simulink model "Model"  (R2021a)
settings: Solver=ode4  StartTime=0.0  StopTime=inf  FixedStep=Ts  RelTol=1e-3
PreLoadFcn:
  | filepath  = fileparts(get_param(bdroot, 'FileName'))
  | cd(filepath);
values from neighbouring files (symbols this model uses):
  A_GRotation = [0 0 0]    [Parameter_PX4.m]
  ACC_UserFault = 0    [Parameter_PX4.m]
  ACCDrift = 0.0    (= 0)    [Parameter_PX4.m]
  ACCNoise = 1.0    (= 1)    [Parameter_PX4.m]
  accnoisegain = 0    [Parameter_PX4.m]
  ACCScale = 1.0    (= 1)    [Parameter_PX4.m]
  BaroNoise = 1.0    (= 1)    [Parameter_PX4.m]
  GyroDrift = 0.0    (= 0)    [Parameter_PX4.m]
  GyroNoise = 1.0    (= 1)    [Parameter_PX4.m]
  GyroScale = 1.0    (= 1)    [Parameter_PX4.m]
  MagDrift = 0.0    (= 0)    [Parameter_PX4.m]
  MagNoise = 1.0    (= 1)    [Parameter_PX4.m]
  MagRotation = [0 0 0]    [Parameter_PX4.m]
  MagScale = 1.0    (= 1)    [Parameter_PX4.m]
  ModelInit_GroundSlope = [0,0]    [Parameter_PX4.m]
  ModelInit_RPM = 0    [Parameter_PX4.m]
  ModelParam_envAltitude = -100    [Parameter_PX4.m]
  ModelParam_GlobalNoiseGainSwitch = 0.4    [Parameter_PX4.m]
  ModelParam_GPSEphFinal = 0.3    [Parameter_PX4.m]
  ModelParam_GPSEpvFinal = 0.4    [Parameter_PX4.m]
  ModelParam_GPSFix3DFix = 3    [Parameter_PX4.m]
  ModelParam_GPSSatsVisible = 10    [Parameter_PX4.m]
  ModelParam_motorCr = 842.1    [Parameter_PX4.m]
  ModelParam_motorJm = 0.0001287    [Parameter_PX4.m]
  ModelParam_motorMinThr = 0.05    [Parameter_PX4.m]
  ModelParam_motorT = 0.0214    [Parameter_PX4.m]
  ModelParam_motorWb = 22.83    [Parameter_PX4.m]
  ModelParam_noiseBaroCoupleWithSpeed = 0    [Parameter_PX4.m]
  ModelParam_noiseUpperWindBodyRatio = 0    [Parameter_PX4.m]
  ModelParam_rotorCm = 2.783e-07    [Parameter_PX4.m]
  ModelParam_rotorCt = 1.681e-05    [Parameter_PX4.m]
  ModelParam_uavCCm = [0.0035 0.0039 0.0034]    [Parameter_PX4.m]
  ModelParam_uavCd = 0.055    [Parameter_PX4.m]
  ModelParam_uavDearo = 0.12    [Parameter_PX4.m]
  ModelParam_uavMass = 1.515    [Parameter_PX4.m]
  ModelParam_uavR = 0.225    [Parameter_PX4.m]
  ModelParam_uavType = int8(3)    [Parameter_PX4.m]
  MyNoiseGain = [2.5;3;4].*3    [Parameter_PX4.m]
  PWMNoiseGain = [10;15;3]    [Parameter_PX4.m]
  TemperatureConstant = 25.0    (= 25)    [Parameter_PX4.m]
  Ts = 1/2000    (= 0.0005)    [Parameter_PX4.m]
  TypeMotorAngMatrix = [     [pi/3 pi -pi/3 0 0 0 0 0];     [pi/3 pi -pi/3 0 0 0 0 0];     [pi/4 pi/4+pi pi/4+3*pi/2 pi/4+pi/2 0 0 0 0];     [pi/2 3*pi/2 0 pi 0 0 0 0];     [pi/2 3/2*pi 3/2*pi+pi/3 pi/2+pi/3 pi/2-pi/3 3/2*pi-pi/3 0 0];     [0 pi pi+pi/3 pi/3 -pi/3 pi-pi/3 0 0];     [pi/3 pi/3 pi pi -pi/3 -pi/3 0 0];     [pi/8 pi+pi/8 pi/8+pi/4 pi-pi/8 -pi/8 3/2*pi-pi/8 3/2*pi+pi/8 pi/2+pi/8];     [0 pi pi/4 3/4*pi -pi/4 ...(+86 chars)    [Parameter_PX4.m]
  TypeMotorDirMatrix = [     [-1 -1 -1 0 0 0 0 0];     [1 1 1 0 0 0 0 0];     [-1 -1 1 1 0 0 0 0];     [-1 -1 1 1 0 0 0 0];     [1 -1 1 -1 -1 1 0 0];     [1 -1 1 -1 -1 1 0 0];     [1 -1 1 -1 1 -1 0 0];     [1 1 -1 -1 -1 -1 1 1];     [1 1 -1 -1 -1 -1 1 1];     [-1 1 -1 1 -1 1 -1 1]; ]'    [Parameter_PX4.m]
  TypeMotorNonVector = int8([3;3;4;4;6;6;6;8;8;8])    [Parameter_PX4.m]
undefined symbols (not defined in the file or in its folder): Earth, ModelParam_GPSEpvInitial, ModelParam_GPSEpvTimeConstant, ModelParam_noiseGPSSampTime, ModelParam_noisePowerIMU, ModelParam_noisePowerOffGainAccel, ModelParam_noisePowerOffGainAccelZ, ModelParam_noisePowerOffGainGyro, ModelParam_noisePowerOffGainGyroZ, ModelParam_noisePowerOffGainMag, ModelParam_noisePowerOffGainMagZ, ModelParam_noisePowerOnGainAccel, ModelParam_noisePowerOnGainAccelZ, ModelParam_noisePowerOnGainGyro, ModelParam_noisePowerOnGainGyroZ, ModelParam_noisePowerOnGainMag, ModelParam_noisePowerOnGainMagZ, ModelParam_noiseUpperGPS, ModelParam_timeSamp, Newton, Raphson, WGS84
libraries: simulink x11, sharedtransform x7, aerolibutil x4, aerolibtransform2 x4, aerolibasang x3, simulink_extras x2, etargetslib x2, aerolibatmos2 x2, shared6dof x1, aerolibconvert2 x1, aerolibobsolete x1, aerolibnav x1
(part 2 of 3)

== system Model/Motor Model/MotorNonlinearDynamic2 ==
  Wb : Inport
  Cr : Inport  Port=2
  motorT : Inport  Port=3
  ModelInit_RPM : Inport  Port=4
  PWM : Inport  Port=5
  Minimum Throttle Cutoff : simulink/Logic and Bit Operations/Compare To Constant  relop=>=  const=ModelParam_motorMinThr  OutDataTypeStr=uint8
  Motor_Dynamics : Subsystem  TreatAsAtomicUnit=on
  Motor_Dynamics_backup : StateSpace  Commented=on  A=-1/ModelParam_motorT  C=1/ModelParam_motorT  D=0  InitialCondition=ModelInit_RPM*ModelParam_motorT
  Product : Product
  Product1 : Product
  Signal_Saturation : Saturate  UpperLimit=0.95  LowerLimit=0
  Sum1 : Sum  Inputs=++|
  radW : Outport  VectorParamsAs1DForOutWhenUnconnected=off
  wires:
  ModelInit_RPM/1 -> Motor_Dynamics/2(ModelInit_RPM)
  motorT/1 -> Motor_Dynamics/3(motorT)
  Cr/1 -> Product1/1
  Minimum Throttle Cutoff/1 -> Product/2
  Wb/1 -> Sum1/1
  Sum1/1 -> Product/1
  Product1/1 -> Sum1/2
  Signal_Saturation/1 -> Minimum Throttle Cutoff/1, Product1/2
  Product/1 -> Motor_Dynamics/1(motor_rate_d)
  Motor_Dynamics/1(motor_rate_act) -> radW/1
  PWM/1 -> Signal_Saturation/1

== system Model/Motor Model/MotorNonlinearDynamic3 ==
  Wb : Inport
  Cr : Inport  Port=2
  motorT : Inport  Port=3
  ModelInit_RPM : Inport  Port=4
  PWM : Inport  Port=5
  Minimum Throttle Cutoff : simulink/Logic and Bit Operations/Compare To Constant  relop=>=  const=ModelParam_motorMinThr  OutDataTypeStr=uint8
  Motor_Dynamics : Subsystem  TreatAsAtomicUnit=on
  Motor_Dynamics_backup : StateSpace  Commented=on  A=-1/ModelParam_motorT  C=1/ModelParam_motorT  D=0  InitialCondition=ModelInit_RPM*ModelParam_motorT
  Product : Product
  Product1 : Product
  Signal_Saturation : Saturate  UpperLimit=0.95  LowerLimit=0
  Sum1 : Sum  Inputs=++|
  radW : Outport  VectorParamsAs1DForOutWhenUnconnected=off
  wires:
  PWM/1 -> Signal_Saturation/1
  Motor_Dynamics/1(motor_rate_act) -> radW/1
  Product/1 -> Motor_Dynamics/1(motor_rate_d)
  Signal_Saturation/1 -> Product1/2, Minimum Throttle Cutoff/1
  Product1/1 -> Sum1/2
  Sum1/1 -> Product/1
  Wb/1 -> Sum1/1
  Minimum Throttle Cutoff/1 -> Product/2
  Cr/1 -> Product1/1
  motorT/1 -> Motor_Dynamics/3(motorT)
  ModelInit_RPM/1 -> Motor_Dynamics/2(ModelInit_RPM)

== system Model/Motor Model/MotorNonlinearDynamic4 ==
  Wb : Inport
  Cr : Inport  Port=2
  motorT : Inport  Port=3
  ModelInit_RPM : Inport  Port=4
  PWM : Inport  Port=5
  Minimum Throttle Cutoff : simulink/Logic and Bit Operations/Compare To Constant  relop=>=  const=ModelParam_motorMinThr  OutDataTypeStr=uint8
  Motor_Dynamics : Subsystem  TreatAsAtomicUnit=on
  Motor_Dynamics_backup : StateSpace  Commented=on  A=-1/ModelParam_motorT  C=1/ModelParam_motorT  D=0  InitialCondition=ModelInit_RPM*ModelParam_motorT
  Product : Product
  Product1 : Product
  Signal_Saturation : Saturate  UpperLimit=0.95  LowerLimit=0
  Sum1 : Sum  Inputs=++|
  radW : Outport  VectorParamsAs1DForOutWhenUnconnected=off
  wires:
  ModelInit_RPM/1 -> Motor_Dynamics/2(ModelInit_RPM)
  motorT/1 -> Motor_Dynamics/3(motorT)
  Cr/1 -> Product1/1
  Minimum Throttle Cutoff/1 -> Product/2
  Wb/1 -> Sum1/1
  Sum1/1 -> Product/1
  Product1/1 -> Sum1/2
  Signal_Saturation/1 -> Minimum Throttle Cutoff/1, Product1/2
  Product/1 -> Motor_Dynamics/1(motor_rate_d)
  Motor_Dynamics/1(motor_rate_act) -> radW/1
  PWM/1 -> Signal_Saturation/1

== system Model/Motor Model/MotorNonlinearDynamic5 ==
  Wb : Inport
  Cr : Inport  Port=2
  motorT : Inport  Port=3
  ModelInit_RPM : Inport  Port=4
  PWM : Inport  Port=5
  Minimum Throttle Cutoff : simulink/Logic and Bit Operations/Compare To Constant  relop=>=  const=ModelParam_motorMinThr  OutDataTypeStr=uint8
  Motor_Dynamics : Subsystem  TreatAsAtomicUnit=on
  Motor_Dynamics_backup : StateSpace  Commented=on  A=-1/ModelParam_motorT  C=1/ModelParam_motorT  D=0  InitialCondition=ModelInit_RPM*ModelParam_motorT
  Product : Product
  Product1 : Product
  Signal_Saturation : Saturate  UpperLimit=0.95  LowerLimit=0
  Sum1 : Sum  Inputs=++|
  radW : Outport  VectorParamsAs1DForOutWhenUnconnected=off
  wires:
  PWM/1 -> Signal_Saturation/1
  Motor_Dynamics/1(motor_rate_act) -> radW/1
  Product/1 -> Motor_Dynamics/1(motor_rate_d)
  Signal_Saturation/1 -> Product1/2, Minimum Throttle Cutoff/1
  Product1/1 -> Sum1/2
  Sum1/1 -> Product/1
  Wb/1 -> Sum1/1
  Minimum Throttle Cutoff/1 -> Product/2
  Cr/1 -> Product1/1
  motorT/1 -> Motor_Dynamics/3(motorT)
  ModelInit_RPM/1 -> Motor_Dynamics/2(ModelInit_RPM)

== system Model/Motor Model/MotorNonlinearDynamic6 ==
  Wb : Inport
  Cr : Inport  Port=2
  motorT : Inport  Port=3
  ModelInit_RPM : Inport  Port=4
  PWM : Inport  Port=5
  Minimum Throttle Cutoff : simulink/Logic and Bit Operations/Compare To Constant  relop=>=  const=ModelParam_motorMinThr  OutDataTypeStr=uint8
  Motor_Dynamics : Subsystem  TreatAsAtomicUnit=on
  Motor_Dynamics_backup : StateSpace  Commented=on  A=-1/ModelParam_motorT  C=1/ModelParam_motorT  D=0  InitialCondition=ModelInit_RPM*ModelParam_motorT
  Product : Product
  Product1 : Product
  Signal_Saturation : Saturate  UpperLimit=0.95  LowerLimit=0
  Sum1 : Sum  Inputs=++|
  radW : Outport  VectorParamsAs1DForOutWhenUnconnected=off
  wires:
  ModelInit_RPM/1 -> Motor_Dynamics/2(ModelInit_RPM)
  motorT/1 -> Motor_Dynamics/3(motorT)
  Cr/1 -> Product1/1
  Minimum Throttle Cutoff/1 -> Product/2
  Wb/1 -> Sum1/1
  Sum1/1 -> Product/1
  Product1/1 -> Sum1/2
  Signal_Saturation/1 -> Minimum Throttle Cutoff/1, Product1/2
  Product/1 -> Motor_Dynamics/1(motor_rate_d)
  Motor_Dynamics/1(motor_rate_act) -> radW/1
  PWM/1 -> Signal_Saturation/1

== system Model/Motor Model/MotorNonlinearDynamic7 ==
  Wb : Inport
  Cr : Inport  Port=2
  motorT : Inport  Port=3
  ModelInit_RPM : Inport  Port=4
  PWM : Inport  Port=5
  Minimum Throttle Cutoff : simulink/Logic and Bit Operations/Compare To Constant  relop=>=  const=ModelParam_motorMinThr  OutDataTypeStr=uint8
  Motor_Dynamics : Subsystem  TreatAsAtomicUnit=on
  Motor_Dynamics_backup : StateSpace  Commented=on  A=-1/ModelParam_motorT  C=1/ModelParam_motorT  D=0  InitialCondition=ModelInit_RPM*ModelParam_motorT
  Product : Product
  Product1 : Product
  Signal_Saturation : Saturate  UpperLimit=0.95  LowerLimit=0
  Sum1 : Sum  Inputs=++|
  radW : Outport  VectorParamsAs1DForOutWhenUnconnected=off
  wires:
  PWM/1 -> Signal_Saturation/1
  Motor_Dynamics/1(motor_rate_act) -> radW/1
  Product/1 -> Motor_Dynamics/1(motor_rate_d)
  Signal_Saturation/1 -> Product1/2, Minimum Throttle Cutoff/1
  Product1/1 -> Sum1/2
  Sum1/1 -> Product/1
  Wb/1 -> Sum1/1
  Minimum Throttle Cutoff/1 -> Product/2
  Cr/1 -> Product1/1
  motorT/1 -> Motor_Dynamics/3(motorT)
  ModelInit_RPM/1 -> Motor_Dynamics/2(ModelInit_RPM)

== system Model/Motor Model/MotorNonlinearDynamic8 ==
  Wb : Inport
  Cr : Inport  Port=2
  motorT : Inport  Port=3
  ModelInit_RPM : Inport  Port=4
  PWM : Inport  Port=5
  Minimum Throttle Cutoff : simulink/Logic and Bit Operations/Compare To Constant  relop=>=  const=ModelParam_motorMinThr  OutDataTypeStr=uint8
  Motor_Dynamics : Subsystem  TreatAsAtomicUnit=on
  Motor_Dynamics_backup : StateSpace  Commented=on  A=-1/ModelParam_motorT  C=1/ModelParam_motorT  D=0  InitialCondition=ModelInit_RPM*ModelParam_motorT
  Product : Product
  Product1 : Product
  Signal_Saturation : Saturate  UpperLimit=0.95  LowerLimit=0
  Sum1 : Sum  Inputs=++|
  radW : Outport  VectorParamsAs1DForOutWhenUnconnected=off
  wires:
  ModelInit_RPM/1 -> Motor_Dynamics/2(ModelInit_RPM)
  motorT/1 -> Motor_Dynamics/3(motorT)
  Cr/1 -> Product1/1
  Minimum Throttle Cutoff/1 -> Product/2
  Wb/1 -> Sum1/1
  Sum1/1 -> Product/1
  Product1/1 -> Sum1/2
  Signal_Saturation/1 -> Minimum Throttle Cutoff/1, Product1/2
  Product/1 -> Motor_Dynamics/1(motor_rate_d)
  Motor_Dynamics/1(motor_rate_act) -> radW/1
  PWM/1 -> Signal_Saturation/1

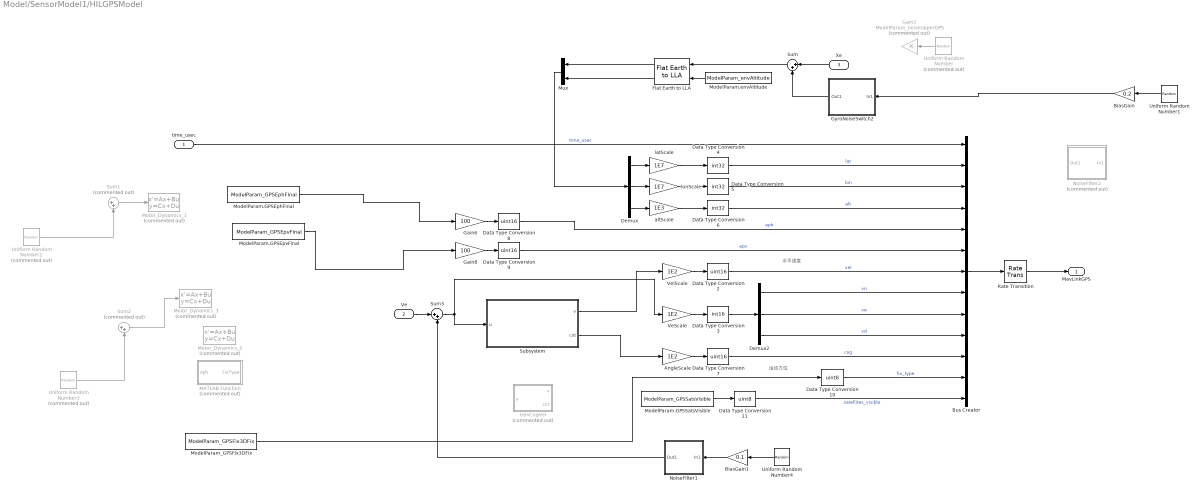
== system Model/SensorModel1/HILGPSModel ==
  note: 水平速度
  note: 运动方位
  time_usec : Inport
  Ve : Inport  Port=2
  Xe : Inport  Port=3
  AngleScale : Gain  Gain=1E2
  BiasGain : Gain  Gain=0.2
  BiasGain1 : Gain  Gain=0.1
  Bus Creator : BusCreator  Inputs=13  OutDataTypeStr=Bus: MavLinkGPS  NonVirtualBus=on
  Data Type Conversion10 : DataTypeConversion  OutDataTypeStr=uint8  RndMeth=Round
  Data Type Conversion11 : DataTypeConversion  OutDataTypeStr=uint8  RndMeth=Round
  Data Type Conversion{2,7..9} (4 alike) : DataTypeConversion  OutDataTypeStr=uint16  RndMeth=Round
  Data Type Conversion3 : DataTypeConversion  OutDataTypeStr=int16  RndMeth=Round
  Data Type Conversion4 : DataTypeConversion  OutDataTypeStr=int32  RndMeth=Round
  Data Type Conversion5 : DataTypeConversion  OutDataTypeStr=int32  RndMeth=Round
  Data Type Conversion6 : DataTypeConversion  OutDataTypeStr=int32  RndMeth=Round
  Demux : Demux  Outputs=3
  Demux2 : Demux  Outputs=3
  Flat Earth to LLA : aerolibtransform2/Flat Earth to LLA  units=Metric (MKS)  ptype=Earth (WGS84)  F=1/298.257223563  R=6378137  refPosPort=off  LL0=ModelParam_GPSLatLong  psi=0
  Gain2 : Gain  Commented=on  Gain=ModelParam_noiseUpperGPS
  Gain6 : Gain  Gain=100
  Gain8 : Gain  Gain=100
  GenCogVel : MATLAB Function  Commented=on  TreatAsAtomicUnit=on
  GyroNoiseSwitch2 : Subsystem
  MATLAB Function : MATLAB Function  Commented=on  TreatAsAtomicUnit=on
  ModelParam.GPSEphFinal : Constant  Value=ModelParam_GPSEphFinal
  ModelParam.GPSEpvFinal : Constant  Value=ModelParam_GPSEpvFinal
  ModelParam.GPSSatsVisible : Constant  Value=ModelParam_GPSSatsVisible
  ModelParam.envAltitude : Constant  Value=ModelParam_envAltitude
  ModelParam_GPSFix3DFix : Constant  Value=ModelParam_GPSFix3DFix
  Motor_Dynamics_1 : StateSpace  Commented=on  A=-1/0.2  C=1/0.2  D=0  InitialCondition=20*0.2
  Motor_Dynamics_2 : StateSpace  Commented=on  A=-1/ModelParam_GPSEpvTimeConstant  C=1/ModelParam_GPSEpvTimeConstant  D=0  InitialCondition=ModelParam_GPSEpvInitial*ModelParam_GPSEpvTimeConstant
  Motor_Dynamics_3 : StateSpace  Commented=on  A=-1/0.2  C=1/0.2  D=0  InitialCondition=20*0.2
  Mux : Mux  Inputs=2
  NoiseFilter1 : Subsystem
  NoiseFilter2 : Subsystem  Commented=on
  Rate Transition : RateTransition  OutPortSampleTime=0.05
  Subsystem : Subsystem
  Sum : Sum  Inputs=|++
  Sum1 : Sum  Commented=on  Inputs=|++
  Sum2 : Sum  Commented=on  Inputs=|++
  Sum3 : Sum  Inputs=|++
  Uniform Random Number : UniformRandomNumber  Commented=on  Minimum=[-1,-1,-3]  Maximum=[1,1,3]  Seed=[14524,7875,698]  SampleTime=ModelParam_timeSamp
  Uniform Random Number1 : UniformRandomNumber  Maximum=[1,1,2]  Seed=[1452,787,69]  SampleTime=0.05
  Uniform Random Number2 : UniformRandomNumber  Commented=on  Minimum=-0.01  Maximum=0.01  Seed=4345454  SampleTime=ModelParam_noiseGPSSampTime
  Uniform Random Number3 : UniformRandomNumber  Commented=on  Seed=3244333  SampleTime=ModelParam_noiseGPSSampTime
  Uniform Random Number4 : UniformRandomNumber  Minimum=[-1,-1,-2]  Maximum=[1,1,2]  Seed=[5445,45433,33433]  SampleTime=0.05
  VeScale : Gain  Gain=1E2
  VelScale : Gain  Gain=1E2
  altScale : Gain  Gain=1E3
  latScale : Gain  Gain=1E7
  lonScale : Gain  Gain=1E7
  MavLinkGPS : Outport  VectorParamsAs1DForOutWhenUnconnected=off
  wires:
  Data Type Conversion8/1 -> Bus Creator/5  "eph"
  Gain8/1 -> Data Type Conversion9/1
  Gain6/1 -> Data Type Conversion8/1
  Data Type Conversion9/1 -> Bus Creator/6  "epv"
  time_usec/1 -> Bus Creator/1  "time_usec"
  latScale/1 -> Data Type Conversion4/1
  lonScale/1 -> Data Type Conversion5/1
  altScale/1 -> Data Type Conversion6/1
  Data Type Conversion4/1 -> Bus Creator/2  "lat"
  Data Type Conversion5/1 -> Bus Creator/3  "lon"
  Data Type Conversion6/1 -> Bus Creator/4  "alt"
  Demux2/1 -> Bus Creator/8  "vn"
  Demux2/2 -> Bus Creator/9  "ve"
  Demux2/3 -> Bus Creator/10  "vd"
  VeScale/1 -> Data Type Conversion3/1
  Data Type Conversion3/1 -> Demux2/1
  VelScale/1 -> Data Type Conversion2/1
  Data Type Conversion2/1 -> Bus Creator/7  "vel"
  AngleScale/1 -> Data Type Conversion7/1
  Data Type Conversion7/1 -> Bus Creator/11  "cog"
  Data Type Conversion11/1 -> Bus Creator/13  "satellites_visible"
  Data Type Conversion10/1 -> Bus Creator/12  "fix_type"
  ModelParam.GPSSatsVisible/1 -> Data Type Conversion11/1
  Flat Earth to LLA/2 -> Mux/2
  ModelParam.envAltitude/1 -> Flat Earth to LLA/2
  Xe/1 -> Sum/1
  Flat Earth to LLA/1 -> Mux/1
  Demux/1 -> latScale/1
  Demux/2 -> lonScale/1
  Demux/3 -> altScale/1
  Uniform Random Number/1 -> Gain2/1
  Sum/1 -> Flat Earth to LLA/1
  Uniform Random Number1/1 -> BiasGain/1
  BiasGain/1 -> GyroNoiseSwitch2/1(In1)
  Mux/1 -> Demux/1
  ModelParam.GPSEphFinal/1 -> Gain6/1
  Sum2/1 -> Motor_Dynamics_3/1
  ModelParam_GPSFix3DFix/1 -> Data Type Conversion10/1
  Ve/1 -> Sum3/1
  GyroNoiseSwitch2/1(Out1) -> Sum/2
  BiasGain1/1 -> NoiseFilter1/1(In1)
  Uniform Random Number4/1 -> BiasGain1/1
  Sum1/1 -> Motor_Dynamics_1/1
  Uniform Random Number2/1 -> Sum1/2
  Uniform Random Number3/1 -> Sum2/2
  ModelParam.GPSEpvFinal/1 -> Gain8/1
  Sum3/1 -> Subsystem/1(u), VeScale/1
  NoiseFilter1/1(Out1) -> Sum3/2
  Subsystem/1(v) -> VelScale/1
  Subsystem/2(cot) -> AngleScale/1
  Bus Creator/1 -> Rate Transition/1
  Rate Transition/1 -> MavLinkGPS/1

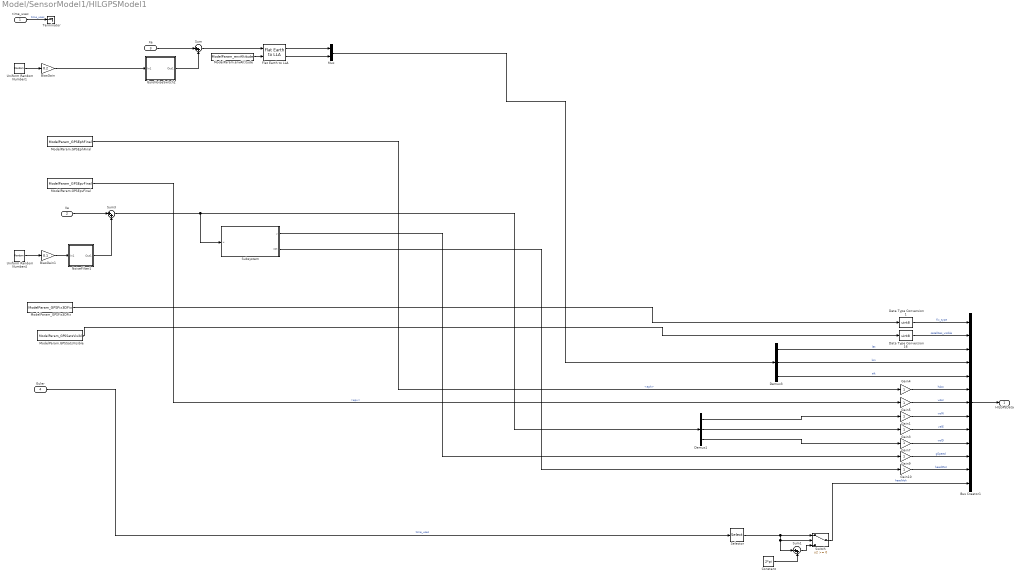
== system Model/SensorModel1/HILGPSModel1 ==
  time_usec : Inport
  Ve : Inport  Port=2
  Xe : Inport  Port=3
  Euler : Inport  Port=4
  BiasGain : Gain  Gain=0.2
  BiasGain1 : Gain  Gain=0.1
  Bus Creator1 : BusCreator  Inputs=13  OutDataTypeStr=Bus: HILGPS  NonVirtualBus=on
  Constant : Constant  Value=2*pi
  Data Type Conversion1 : DataTypeConversion  OutDataTypeStr=uint8  RndMeth=Round
  Data Type Conversion16 : DataTypeConversion  OutDataTypeStr=uint8  RndMeth=Round
  Demux1 : Demux  Outputs=3
  Demux3 : Demux  Outputs=3
  Flat Earth to LLA : aerolibtransform2/Flat Earth to LLA  units=Metric (MKS)  ptype=Earth (WGS84)  F=1/298.257223563  R=6378137  refPosPort=off  LL0=ModelParam_GPSLatLong  psi=0
  Gain{1,3..5,7,9..10} (7 alike) : Gain
  GyroNoiseSwitch2 : Subsystem
  ModelParam.GPSEphFinal : Constant  Value=ModelParam_GPSEphFinal
  ModelParam.GPSEpvFinal : Constant  Value=ModelParam_GPSEpvFinal
  ModelParam.GPSSatsVisible : Constant  Value=ModelParam_GPSSatsVisible
  ModelParam.envAltitude : Constant  Value=ModelParam_envAltitude
  ModelParam_GPSFix3DFix : Constant  Value=ModelParam_GPSFix3DFix
  Mux : Mux  Inputs=2
  NoiseFilter1 : Subsystem
  Selector : Selector  IndexMode=Zero-based  InputPortWidth=3  IndexOptions=Index vector (dialog)  Indices=[2]  OutputSizes=1
  Subsystem : Subsystem
  Sum : Sum  Inputs=|++
  Sum1 : Sum  Inputs=|++
  Sum3 : Sum  Inputs=|++
  Switch : Switch
  Terminator : Terminator
  Uniform Random Number1 : UniformRandomNumber  Minimum=[-1,-1,-2]  Maximum=[1,1,2]  Seed=[1452,787,69]  SampleTime=Ts
  Uniform Random Number4 : UniformRandomNumber  Minimum=[-1,-1,-2]  Maximum=[1,1,2]  Seed=[5445,45433,33433]  SampleTime=Ts
  HILGPSData : Outport  VectorParamsAs1DForOutWhenUnconnected=off
  wires:
  ModelParam.GPSSatsVisible/1 -> Data Type Conversion16/1
  Flat Earth to LLA/2 -> Mux/2
  ModelParam.envAltitude/1 -> Flat Earth to LLA/2
  Xe/1 -> Sum/1
  Flat Earth to LLA/1 -> Mux/1
  Sum/1 -> Flat Earth to LLA/1
  Uniform Random Number1/1 -> BiasGain/1
  BiasGain/1 -> GyroNoiseSwitch2/1(In1)
  Mux/1 -> Demux3/1
  ModelParam_GPSFix3DFix/1 -> Data Type Conversion1/1
  Ve/1 -> Sum3/1
  GyroNoiseSwitch2/1(Out1) -> Sum/2
  BiasGain1/1 -> NoiseFilter1/1(In1)
  Uniform Random Number4/1 -> BiasGain1/1
  Sum3/1 -> Subsystem/1(u), Demux1/1
  NoiseFilter1/1(Out1) -> Sum3/2
  Gain9/1 -> Bus Creator1/11  "gSpeed"
  Gain1/1 -> Bus Creator1/8  "velN"
  Demux1/1 -> Gain1/1
  Gain7/1 -> Bus Creator1/10  "velD"
  Gain3/1 -> Bus Creator1/9  "velE"
  Gain10/1 -> Bus Creator1/12  "headMot"
  Demux1/2 -> Gain3/1
  ModelParam.GPSEpvFinal/1 -> Gain5/1  "<epv>"
  ModelParam.GPSEphFinal/1 -> Gain4/1  "<eph>"
  Demux1/3 -> Gain7/1
  Gain5/1 -> Bus Creator1/7  "vAcc"
  Subsystem/1(v) -> Gain9/1
  Subsystem/2(cot) -> Gain10/1
  Gain4/1 -> Bus Creator1/6  "hAcc"
  Data Type Conversion16/1 -> Bus Creator1/2  "satellites_visible"
  Data Type Conversion1/1 -> Bus Creator1/1  "fix_type"
  Bus Creator1/1 -> HILGPSData/1
  Switch/1 -> Bus Creator1/13  "headVeh"
  Selector/1 -> Switch/1, Switch/2, Sum1/1
  Euler/1 -> Selector/1  "time_usec"
  Demux3/1 -> Bus Creator1/3  "lat"
  Demux3/2 -> Bus Creator1/4  "lon"
  Demux3/3 -> Bus Creator1/5  "alt"
  Constant/1 -> Sum1/2
  Sum1/1 -> Switch/3
  time_usec/1 -> Terminator/1  "time_usec"

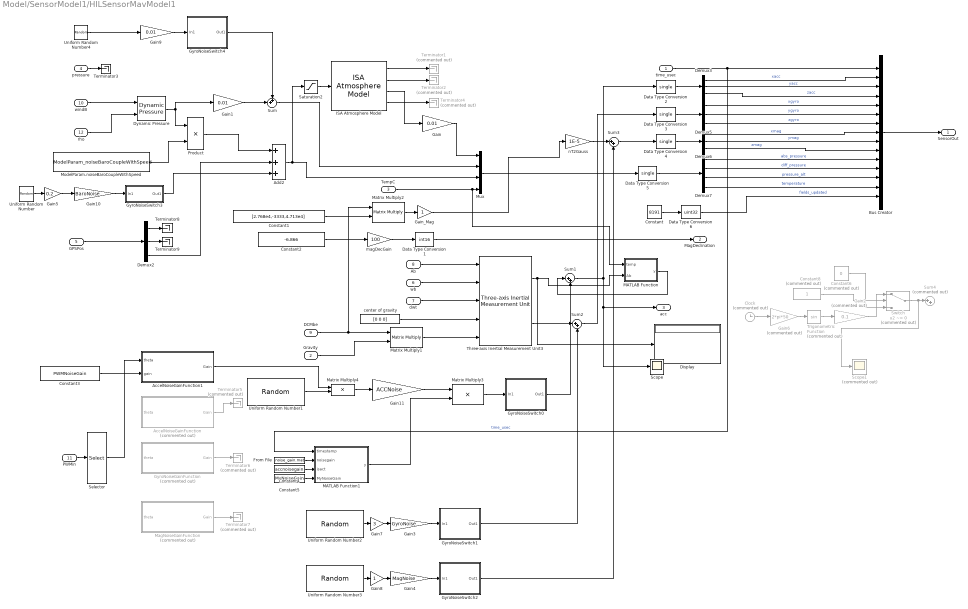
== system Model/SensorModel1/HILSensorMavModel1 ==
  time_usec : Inport
  Gravity : Inport  Port=2
  TempC : Inport  Port=3
  pressure : Inport  Port=4
  GPSPos : Inport  Port=5
  wb : Inport  Port=6
  dwt : Inport  Port=7
  Ab : Inport  Port=8
  DCMbe : Inport  Port=9
  windB : Inport  Port=10
  PWMin : Inport  Port=11
  rho : Inport  Port=12
  AccelNoiseGainFunction : MATLAB Function  Commented=on  TreatAsAtomicUnit=on
  AccelNoiseGainFunction1 : MATLAB Function  TreatAsAtomicUnit=on
  Add2 : Sum  Inputs=+++
  Bus Creator : BusCreator  Inputs=15  OutDataTypeStr=Bus: MavLinkSensor  NonVirtualBus=on
  Clock : Clock  Commented=on
  Constant : Constant  Value=8191
  Constant1 : Constant  Value=[2.768e4,-3333,4.713e4]
  Constant2 : Constant  Value=-6.866
  Constant3 : Constant  Value=PWMNoiseGain
  Constant4 : Constant  Value=accnoisegain
  Constant5 : Constant  Value=MyNoiseGain
  Constant6 : Constant  Commented=on  Value=0
  Constant8 : Constant  Commented=on  OutDataTypeStr=uint8
  Data Type Conversion1 : DataTypeConversion  OutDataTypeStr=int16
  Data Type Conversion{2..5} (4 alike) : DataTypeConversion  OutDataTypeStr=single
  Data Type Conversion6 : DataTypeConversion  OutDataTypeStr=uint32
  Demux{2..3,5..6} (4 alike) : Demux  Outputs=3
  Demux7 : Demux
  Display : Display
  Dynamic Pressure : aerolibasang/Dynamic Pressure
  From File : FromFile  FileName=noise_gain.mat  SampleTime=0
  Gain : Gain  Gain=0.01
  Gain1 : Gain  Gain=0.01
  Gain10 : Gain  Gain=BaroNoise
  Gain11 : Gain  Gain=ACCNoise
  Gain2 : Gain  Commented=on  Gain=0.1
  Gain3 : Gain  Gain=GyroNoise
  Gain4 : Gain  Gain=MagNoise
  Gain5 : Gain  Gain=0.2
  Gain6 : Gain  Commented=on  Gain=2*pi*50
  Gain7 : Gain  Gain=3
  Gain8 : Gain
  Gain9 : Gain  Gain=0.01
  Gain_Mag : Gain
  GyroNoiseGainFunction : MATLAB Function  Commented=on  TreatAsAtomicUnit=on
  GyroNoiseSwitch0 : Subsystem
  GyroNoiseSwitch1 : Subsystem
  GyroNoiseSwitch2 : Subsystem
  GyroNoiseSwitch3 : Subsystem
  GyroNoiseSwitch4 : Subsystem
  ISA Atmosphere Model : aerolibatmos2/ISA Atmosphere Model  custom=off  g=9.80665  gamma=1.4  R=287.0531  L=0.0065  h_trop=11000  h_strat=20000  rho0=1.225  P0=101325  T0=288.15  h0=0
  MATLAB Function : MATLAB Function  TreatAsAtomicUnit=on
  MATLAB Function1 : MATLAB Function  TreatAsAtomicUnit=on
  MagNoiseGainFunction : MATLAB Function  Commented=on  TreatAsAtomicUnit=on
  Matrix Multiply1 : Product  Multiplication=Matrix(*)
  Matrix Multiply2 : Product  Multiplication=Matrix(*)
  Matrix Multiply3 : Product
  Matrix Multiply4 : Product
  ModelParam.noiseBaroCoupleWithSpeed : Constant  Value=ModelParam_noiseBaroCoupleWithSpeed
  Mux : Mux
  Product : Product
  Saturation2 : Saturate  UpperLimit=100000  LowerLimit=0
  Scope : Scope
  Scope1 : Scope  Commented=on
  Selector : Selector  InputPortWidth=8  IndexOptions=Index vector (dialog)  Indices=[1]  OutputSizes=1
  Sum : Sum  Inputs=++|
  Sum1 : Sum  Inputs=|++
  Sum2 : Sum  Inputs=|++
  Sum3 : Sum  Inputs=|++
  Sum4 : Sum  Commented=on  Inputs=|++
  Switch : Switch  Commented=on  Criteria=u2 ~= 0
  Terminator{1..2,4..7} (6 alike) : Terminator  Commented=on
  Terminator3 : Terminator
  Terminator8 : Terminator
  Terminator9 : Terminator
  Three-axis Inertial Measurement Unit3 : aerolibnav/Three-axis Inertial Measurement Unit  units=Metric (MKS)  imu=[0 0 0]  i_Ts=0  dtype_a=on  w_a=190  z_a=0.707  a_sf_cc=[1 0 0; 0 1 0; 0 0 1]  a_bias=ACC_bias  a_sat="[-160  -160  -160 160 160 160]"  dtype_g=on  w_g=190  z_g=0.707  g_sf_cc=[1 0 0; 0 1 0; 0 0 1]  g_bias=[0 0 0]  g_sens=Gyro_bias  g_sat="[-4.36  -4.36  -4.36 4.36 4.36 4.36]"  i_rand=off  i_seeds=[23093 23094 23095 23096 23097 23098]  i_pow=ModelParam_noisePowerIMU*[0.0000005 0.0000005 0.0000005 0.000000002 0.000000002 0.000000002]
  Trigonometric Function : Trigonometry  Commented=on
  Uniform Random Number : UniformRandomNumber  Minimum=-2  Maximum=2  Seed=15634  SampleTime=0.01
  Uniform Random Number1 : UniformRandomNumber  Minimum=-[0.1,0.1,0.1]  Maximum=[0.1,0.1,0.1]  Seed=[12233,645554,678766]  SampleTime=0.004
  Uniform Random Number2 : UniformRandomNumber  Minimum=-[0.01,0.01,0.01]  Maximum=[0.01,0.01,0.01]  Seed=[3243,44556,2334343]  SampleTime=0.004
  Uniform Random Number3 : UniformRandomNumber  Minimum=-[0.01,0.01,0.01]  Maximum=[0.01,0.01,0.01]  Seed=[45465,454534,1234232]  SampleTime=0.004
  Uniform Random Number4 : UniformRandomNumber  Seed=25634  SampleTime=0.01
  center of gravity : Constant  Value=[0 0 0]
  magDecGain : Gain  Gain=100
  nT2Gauss : Gain  Gain=1E-5
  SensorOut : Outport  VectorParamsAs1DForOutWhenUnconnected=off
  MagDeclination : Outport  Port=2  VectorParamsAs1DForOutWhenUnconnected=off
  acc : Outport  Port=3  VectorParamsAs1DForOutWhenUnconnected=off
  wires:
  center of gravity/1 -> Three-axis Inertial Measurement Unit3/4
  Sum1/1 -> Scope/1, acc/1, Data Type Conversion2/1
  Sum2/1 -> Data Type Conversion3/1
  Sum3/1 -> Data Type Conversion4/1
  Matrix Multiply2/1 -> Gain_Mag/1
  magDecGain/1 -> Data Type Conversion1/1
  GyroNoiseSwitch3/1(Out1) -> Add2/3
  Product/1 -> Add2/1
  ModelParam.noiseBaroCoupleWithSpeed/1 -> Product/2
  rho/1 -> Dynamic Pressure/2
  windB/1 -> Dynamic Pressure/1
  dwt/1 -> Three-axis Inertial Measurement Unit3/3
  Gain_Mag/1 -> nT2Gauss/1
  Dynamic Pressure/1 -> Gain1/1, Product/1
  pressure/1 -> Terminator3/1
  Add2/1 -> Mux/3, Saturation2/1
  Matrix Multiply1/1 -> Three-axis Inertial Measurement Unit3/5
  DCMbe/1 -> Matrix Multiply2/1, Matrix Multiply1/1
  Gravity/1 -> Matrix Multiply1/2
  Sum/1 -> Mux/2
  Gain/1 -> Mux/1
  Data Type Conversion6/1 -> Bus Creator/15  "fields_updated"
  Constant/1 -> Data Type Conversion6/1
  time_usec/1 -> MATLAB Function1/1(timestamp), Bus Creator/1  "time_usec"
  Demux7/2 -> Bus Creator/12  "diff_pressure"
  Demux7/3 -> Bus Creator/13  "pressure_alt"
  Demux6/2 -> Bus Creator/9  "ymag"
  Demux6/3 -> Bus Creator/10  "zmag"
  TempC/1 -> MATLAB Function/1(temp), Mux/4
  Demux7/1 -> Bus Creator/11  "abs_pressure"
  Demux5/2 -> Bus Creator/6  "ygyro"
  Demux6/1 -> Bus Creator/8  "xmag"
  Demux5/3 -> Bus Creator/7  "zgyro"
  Demux7/4 -> Bus Creator/14  "temperature"
  Demux3/1 -> Bus Creator/2  "xacc"
  Demux3/2 -> Bus Creator/3  "yacc"
  Demux5/1 -> Bus Creator/5  "xgyro"
  Demux3/3 -> Bus Creator/4  "zacc"
  PWMin/1 -> Selector/1
  wb/1 -> Three-axis Inertial Measurement Unit3/2
  AccelNoiseGainFunction/1(Gain) -> Terminator5/1
  nT2Gauss/1 -> Sum3/1
  GyroNoiseSwitch1/1(Out1) -> Sum2/2
  GyroNoiseSwitch2/1(Out1) -> Sum3/2
  Data Type Conversion2/1 -> Demux3/1
  Data Type Conversion3/1 -> Demux5/1
  Data Type Conversion4/1 -> Demux6/1
  Data Type Conversion5/1 -> Demux7/1
  Bus Creator/1 -> SensorOut/1
  Data Type Conversion1/1 -> MagDeclination/1
  Three-axis Inertial Measurement Unit3/2 -> Sum2/1
  ISA Atmosphere Model/2 -> Terminator2/1
  ISA Atmosphere Model/4 -> Terminator4/1
  ISA Atmosphere Model/1 -> Terminator1/1
  Gain10/1 -> GyroNoiseSwitch3/1(In1)
  GyroNoiseSwitch0/1(Out1) -> Sum1/2
  GyroNoiseGainFunction/1(Gain) -> Terminator6/1
  MagNoiseGainFunction/1(Gain) -> Terminator7/1
  ISA Atmosphere Model/3 -> Gain/1
  Gain9/1 -> GyroNoiseSwitch4/1(In1)
  Uniform Random Number4/1 -> Gain9/1
  Gain1/1 -> Sum/2
  GyroNoiseSwitch4/1(Out1) -> Sum/1
  Saturation2/1 -> ISA Atmosphere Model/1
  Constant2/1 -> magDecGain/1
  Constant1/1 -> Matrix Multiply2/2
  Mux/1 -> Data Type Conversion5/1
  GPSPos/1 -> Demux2/1
  Demux2/3 -> Add2/2
  Demux2/1 -> Terminator8/1
  Demux2/2 -> Terminator9/1
  Uniform Random Number2/1 -> Gain7/1
  Gain8/1 -> Gain4/1
  Uniform Random Number3/1 -> Gain8/1
  Gain7/1 -> Gain3/1
  Gain3/1 -> GyroNoiseSwitch1/1(In1)
  Gain4/1 -> GyroNoiseSwitch2/1(In1)
  Uniform Random Number/1 -> Gain5/1
  Gain5/1 -> Gain10/1
  Ab/1 -> Three-axis Inertial Measurement Unit3/1
  From File/1 -> MATLAB Function1/2(noisegain)
  Constant4/1 -> MATLAB Function1/3(isact)
  Selector/1 -> AccelNoiseGainFunction1/1(theta)
  AccelNoiseGainFunction1/1(Gain) -> Matrix Multiply4/1
  Uniform Random Number1/1 -> Matrix Multiply4/2
  Constant3/1 -> AccelNoiseGainFunction1/2(gain)
  Matrix Multiply3/1 -> GyroNoiseSwitch0/1(In1)
  Constant5/1 -> MATLAB Function1/4(MyNoiseGain)
  MATLAB Function1/1(y) -> Matrix Multiply3/2
  Trigonometric Function/1 -> Gain2/1
  Switch/1 -> Scope1/1, Sum4/1
  Constant8/1 -> Switch/2
  Gain2/1 -> Switch/1
  Constant6/1 -> Switch/3
  Gain6/1 -> Trigonometric Function/1
  Clock/1 -> Gain6/1
  Matrix Multiply4/1 -> Gain11/1
  Gain11/1 -> Matrix Multiply3/1
  Three-axis Inertial Measurement Unit3/1 -> Display/1, MATLAB Function/2(Ab)
  MATLAB Function/1(y) -> Sum1/1

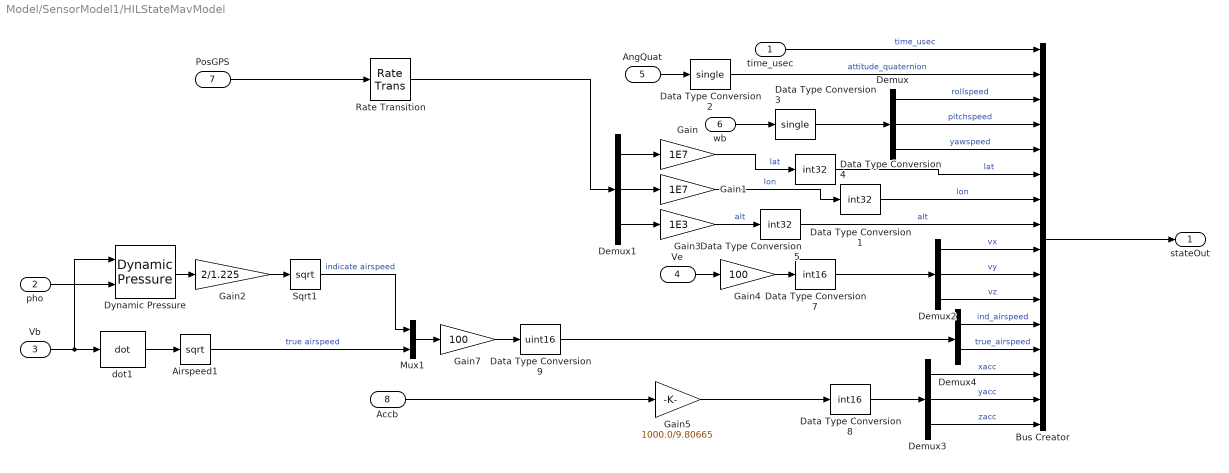
== system Model/SensorModel1/HILStateMavModel ==
  time_usec : Inport
  pho : Inport  Port=2
  Vb : Inport  Port=3
  Ve : Inport  Port=4
  AngQuat : Inport  Port=5
  wb : Inport  Port=6
  PosGPS : Inport  Port=7
  Accb : Inport  Port=8
  Airspeed1 : Sqrt  AlgorithmType=Newton-Raphson  SaturateOnIntegerOverflow=on
  Bus Creator : BusCreator  Inputs=16  OutDataTypeStr=Bus: MavLinkStateQuat  NonVirtualBus=on
  Data Type Conversion1 : DataTypeConversion  OutDataTypeStr=int32  RndMeth=Round
  Data Type Conversion2 : DataTypeConversion  OutDataTypeStr=single
  Data Type Conversion3 : DataTypeConversion  OutDataTypeStr=single
  Data Type Conversion4 : DataTypeConversion  OutDataTypeStr=int32  RndMeth=Round
  Data Type Conversion5 : DataTypeConversion  OutDataTypeStr=int32  RndMeth=Round
  Data Type Conversion7 : DataTypeConversion  OutDataTypeStr=int16  RndMeth=Round
  Data Type Conversion8 : DataTypeConversion  OutDataTypeStr=int16  RndMeth=Round
  Data Type Conversion9 : DataTypeConversion  OutDataTypeStr=uint16  RndMeth=Round
  Demux{,1..3} (4 alike) : Demux  Outputs=3
  Demux4 : Demux  Outputs=2
  Dynamic Pressure : aerolibasang/Dynamic Pressure
  Gain : Gain  Gain=1E7
  Gain1 : Gain  Gain=1E7
  Gain2 : Gain  Gain=2/1.225
  Gain3 : Gain  Gain=1E3
  Gain4 : Gain  Gain=100
  Gain5 : Gain  Gain=1000.0/9.80665
  Gain7 : Gain  Gain=100
  Mux1 : Mux  Inputs=2
  Rate Transition : RateTransition  InitialCondition=[0,0,0]
  Sqrt1 : Sqrt  SaturateOnIntegerOverflow=on
  dot1 : aerolibasang/Incidence, Sideslip, & Airspeed/dot  SystemSampleTime=-1  VariantActivationTime=update diagram  Latency=0  AutoFrameSizeCalculation=off
      settings: SourceProductBaseCode=AE
  stateOut : Outport  VectorParamsAs1DForOutWhenUnconnected=off
  wires:
  Sqrt1/1 -> Mux1/1  "indicate airspeed"
  Gain2/1 -> Sqrt1/1
  Dynamic Pressure/1 -> Gain2/1
  time_usec/1 -> Bus Creator/1  "time_usec"
  Vb/1 -> dot1/1, Dynamic Pressure/1
  AngQuat/1 -> Data Type Conversion2/1
  Ve/1 -> Gain4/1
  wb/1 -> Data Type Conversion3/1
  Airspeed1/1 -> Mux1/2  "true airspeed"
  Mux1/1 -> Gain7/1
  Demux4/1 -> Bus Creator/12  "ind_airspeed"
  Demux4/2 -> Bus Creator/13  "true_airspeed"
  Demux3/3 -> Bus Creator/16  "zacc"
  Demux3/2 -> Bus Creator/15  "yacc"
  Demux3/1 -> Bus Creator/14  "xacc"
  Gain5/1 -> Data Type Conversion8/1
  Accb/1 -> Gain5/1
  Demux2/3 -> Bus Creator/11  "vz"
  Demux2/2 -> Bus Creator/10  "vy"
  Demux2/1 -> Bus Creator/9  "vx"
  Gain4/1 -> Data Type Conversion7/1
  Gain3/1 -> Data Type Conversion5/1  "alt"
  Gain1/1 -> Data Type Conversion1/1  "lon"
  Gain/1 -> Data Type Conversion4/1  "lat"
  Demux1/3 -> Gain3/1
  Demux1/2 -> Gain1/1
  Demux1/1 -> Gain/1
  Demux/3 -> Bus Creator/5  "yawspeed"
  Demux/2 -> Bus Creator/4  "pitchspeed"
  Demux/1 -> Bus Creator/3  "rollspeed"
  Data Type Conversion2/1 -> Bus Creator/2  "attitude_quaternion"
  pho/1 -> Dynamic Pressure/2
  Gain7/1 -> Data Type Conversion9/1
  dot1/1 -> Airspeed1/1
  Data Type Conversion3/1 -> Demux/1
  Data Type Conversion7/1 -> Demux2/1
  Data Type Conversion9/1 -> Demux4/1
  Data Type Conversion8/1 -> Demux3/1
  Data Type Conversion4/1 -> Bus Creator/6  "lat"
  Data Type Conversion1/1 -> Bus Creator/7  "lon"
  Data Type Conversion5/1 -> Bus Creator/8  "alt"
  Bus Creator/1 -> stateOut/1
  PosGPS/1 -> Rate Transition/1
  Rate Transition/1 -> Demux1/1

== system Model/Force and Moment Model/Ground Model New/If Action Subsystem ==
  mg3 : Inport
  ve3 : Inport  Port=2
  Action Port : ActionPort  ActionPortLabel=if(u1 < 0.05)
  Gain : Gain  Gain=-1
  Gain1 : Gain  Gain=-10
  Sum : Sum  Inputs=|++
  F13 : Outport  VectorParamsAs1DForOutWhenUnconnected=off
  wires:
  mg3/1 -> Gain/1
  ve3/1 -> Gain1/1
  Gain/1 -> Sum/1
  Gain1/1 -> Sum/2
  Sum/1 -> F13/1

== system Model/Force and Moment Model/Ground Model New/If Action Subsystem1 ==
  mg3 : Inport
  ve3 : Inport  Port=2
  z : Inport  Port=3
  Action Port : ActionPort  ActionPortLabel=elseif(u1<0.1)
  Gain : Gain  Gain=-1
  Gain1 : Gain  Gain=-10
  Gain2 : Gain  Gain=-0.5
  Sum : Sum  Inputs=+++
  F13 : Outport  VectorParamsAs1DForOutWhenUnconnected=off
  wires:
  Gain1/1 -> Sum/2
  ve3/1 -> Gain1/1
  Sum/1 -> F13/1
  Gain/1 -> Sum/1
  mg3/1 -> Gain/1
  z/1 -> Gain2/1
  Gain2/1 -> Sum/3

== system Model/Force and Moment Model/Ground Model New/If Action Subsystem2 ==
  mg3 : Inport
  ve3 : Inport  Port=2
  z : Inport  Port=3
  Action Port : ActionPort  ActionPortLabel=else
  Gain : Gain  Gain=-1
  Gain1 : Gain  Gain=-50
  Gain2 : Gain  Gain=-1
  Sum : Sum  Inputs=+++
  F13 : Outport  VectorParamsAs1DForOutWhenUnconnected=off
  wires:
  mg3/1 -> Gain/1
  ve3/1 -> Gain1/1
  Gain1/1 -> Sum/2
  Gain/1 -> Sum/1
  Gain2/1 -> Sum/3
  Sum/1 -> F13/1
  z/1 -> Gain2/1

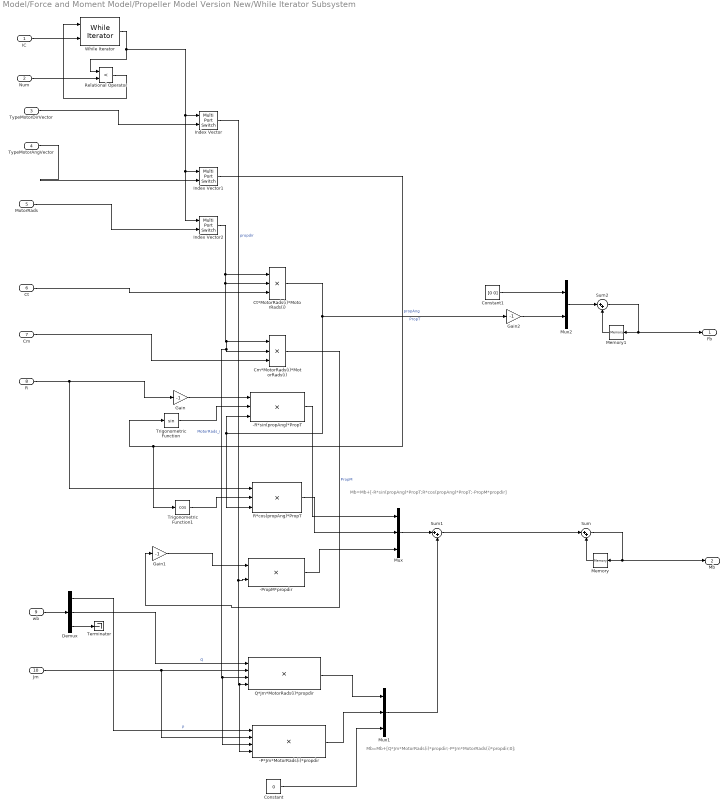
== system Model/Force and Moment Model/Propeller Model Version New/While Iterator Subsystem ==
  note: Mb=Mb+[Q*Jm*MotorRads(i)*propdir;-P*Jm*MotorRads(i)*propdir;0];
  note: Mb=Mb+[-R*sin(propAng)*PropT;R*cos(propAng)*PropT;-PropM*propdir]
  IC : Inport
  Num : Inport  Port=2
  TypeMotorDirVector : Inport  Port=3
  TypeMotorAngVector : Inport  Port=4
  MotorRads : Inport  Port=5
  Ct : Inport  Port=6
  Cm : Inport  Port=7
  R : Inport  Port=8
  wb : Inport  Port=9
  Jm : Inport  Port=10
  -P*Jm*MotorRads(i)*propdir : Product  Inputs=****
  -PropM*propdir : Product  Inputs=**
  -R*sin(propAng)*PropT : Product  Inputs=***
  Cm*MotorRads(i)*MotorRads(i) : Product  Inputs=***
  Constant : Constant  Value=0
  Constant1 : Constant  Value=[0 0]
  Ct*MotorRads(i)*MotorRads(i) : Product  Inputs=***
  Demux : Demux  Outputs=3
  Gain : Gain  Gain=-1
  Gain1 : Gain  Gain=-1
  Gain2 : Gain  Gain=-1
  Index Vector : MultiPortSwitch  Inputs=1
  Index Vector1 : MultiPortSwitch  Inputs=1
  Index Vector2 : MultiPortSwitch  Inputs=1
  Memory : Memory  InitialCondition=[0,0,0]  InheritSampleTime=on
  Memory1 : Memory  InitialCondition=[0,0,0]  InheritSampleTime=on
  Mux : Mux  Inputs=3
  Mux1 : Mux  Inputs=3
  Mux2 : Mux  Inputs=2
  Q*Jm*MotorRads(i)*propdir : Product  Inputs=****
  R*cos(propAng)*PropT : Product  Inputs=***
  Relational Operator : RelationalOperator  Operator=<  OutDataTypeStr=boolean  RndMeth=Simplest
  Sum : Sum  Inputs=|++
  Sum1 : Sum  Inputs=|++
  Sum2 : Sum  Inputs=|++
  Terminator : Terminator
  Trigonometric Function : Trigonometry
  Trigonometric Function1 : Trigonometry  Operator=cos
  While Iterator : WhileIterator  MaxIters=8  ResetStates=reset  ShowIterationPort=on
  Fb : Outport  VectorParamsAs1DForOutWhenUnconnected=off
  Mb : Outport  Port=2  VectorParamsAs1DForOutWhenUnconnected=off
  wires:
  IC/1 -> While Iterator/2
  While Iterator/1 -> Index Vector/1, Index Vector2/1, Index Vector1/1, Relational Operator/1
  Sum/1 -> Memory/1, Mb/1
  Memory/1 -> Sum/2
  Num/1 -> Relational Operator/2
  Relational Operator/1 -> While Iterator/1
  TypeMotorDirVector/1 -> Index Vector/2
  TypeMotorAngVector/1 -> Index Vector1/2
  MotorRads/1 -> Index Vector2/2
  Index Vector/1 -> -PropM*propdir/2, -P*Jm*MotorRads(i)*propdir/4, Q*Jm*MotorRads(i)*propdir/4  "propdir"
  Index Vector1/1 -> Trigonometric Function1/1, Trigonometric Function/1  "propAng"
  Index Vector2/1 -> -P*Jm*MotorRads(i)*propdir/3, Q*Jm*MotorRads(i)*propdir/3, Cm*MotorRads(i)*MotorRads(i)/2, Cm*MotorRads(i)*MotorRads(i)/1, Ct*MotorRads(i)*MotorRads(i)/2, Ct*MotorRads(i)*MotorRads(i)/1  "MotorRads_i"
  Ct/1 -> Ct*MotorRads(i)*MotorRads(i)/3
  Ct*MotorRads(i)*MotorRads(i)/1 -> Gain2/1, R*cos(propAng)*PropT/3, -R*sin(propAng)*PropT/3  "PropT"
  Cm/1 -> Cm*MotorRads(i)*MotorRads(i)/3
  Cm*MotorRads(i)*MotorRads(i)/1 -> Gain1/1  "PropM"
  Gain/1 -> -R*sin(propAng)*PropT/1
  Trigonometric Function/1 -> -R*sin(propAng)*PropT/2
  Trigonometric Function1/1 -> R*cos(propAng)*PropT/2
  R/1 -> R*cos(propAng)*PropT/1, Gain/1
  Gain1/1 -> -PropM*propdir/1
  -R*sin(propAng)*PropT/1 -> Mux/1
  R*cos(propAng)*PropT/1 -> Mux/2
  -PropM*propdir/1 -> Mux/3
  wb/1 -> Demux/1
  Demux/1 -> -P*Jm*MotorRads(i)*propdir/1  "P"
  Demux/2 -> Q*Jm*MotorRads(i)*propdir/1  "Q"
  Jm/1 -> -P*Jm*MotorRads(i)*propdir/2, Q*Jm*MotorRads(i)*propdir/2
  Q*Jm*MotorRads(i)*propdir/1 -> Mux1/1
  -P*Jm*MotorRads(i)*propdir/1 -> Mux1/2
  Constant/1 -> Mux1/3
  Mux/1 -> Sum1/1
  Mux1/1 -> Sum1/2
  Sum1/1 -> Sum/1
  Demux/3 -> Terminator/1
  Gain2/1 -> Mux2/2
  Constant1/1 -> Mux2/1
  Memory1/1 -> Sum2/2
  Sum2/1 -> Memory1/1, Fb/1
  Mux2/1 -> Sum2/1

== system Model/Motor Model/MotorNonlinearDynamic1/Motor_Dynamics ==
  motor_rate_d : Inport
  ModelInit_RPM : Inport  Port=2
  motorT : Inport  Port=3
  Add : Sum  Inputs=+-
  Divide : Product  Inputs=*/
  Integrator : Integrator  InitialConditionSource=external
  motor_rate_act : Outport  VectorParamsAs1DForOutWhenUnconnected=off
  wires:
  motorT/1 -> Divide/2
  Integrator/1 -> Add/2, motor_rate_act/1  "x"
  Divide/1 -> Integrator/1  "drate/dt"
  motor_rate_d/1 -> Add/1
  ModelInit_RPM/1 -> Integrator/2
  Add/1 -> Divide/1

== system Model/Motor Model/MotorNonlinearDynamic2/Motor_Dynamics ==
  motor_rate_d : Inport
  ModelInit_RPM : Inport  Port=2
  motorT : Inport  Port=3
  Add : Sum  Inputs=+-
  Divide : Product  Inputs=*/
  Integrator : Integrator  InitialConditionSource=external
  motor_rate_act : Outport  VectorParamsAs1DForOutWhenUnconnected=off
  wires:
  Add/1 -> Divide/1
  ModelInit_RPM/1 -> Integrator/2
  motor_rate_d/1 -> Add/1
  Divide/1 -> Integrator/1  "drate/dt"
  Integrator/1 -> motor_rate_act/1, Add/2  "x"
  motorT/1 -> Divide/2

== system Model/Motor Model/MotorNonlinearDynamic3/Motor_Dynamics ==
  motor_rate_d : Inport
  ModelInit_RPM : Inport  Port=2
  motorT : Inport  Port=3
  Add : Sum  Inputs=+-
  Divide : Product  Inputs=*/
  Integrator : Integrator  InitialConditionSource=external
  motor_rate_act : Outport  VectorParamsAs1DForOutWhenUnconnected=off
  wires:
  motorT/1 -> Divide/2
  Integrator/1 -> Add/2, motor_rate_act/1  "x"
  Divide/1 -> Integrator/1  "drate/dt"
  motor_rate_d/1 -> Add/1
  ModelInit_RPM/1 -> Integrator/2
  Add/1 -> Divide/1

== system Model/Motor Model/MotorNonlinearDynamic4/Motor_Dynamics ==
  motor_rate_d : Inport
  ModelInit_RPM : Inport  Port=2
  motorT : Inport  Port=3
  Add : Sum  Inputs=+-
  Divide : Product  Inputs=*/
  Integrator : Integrator  InitialConditionSource=external
  motor_rate_act : Outport  VectorParamsAs1DForOutWhenUnconnected=off
  wires:
  Add/1 -> Divide/1
  ModelInit_RPM/1 -> Integrator/2
  motor_rate_d/1 -> Add/1
  Divide/1 -> Integrator/1  "drate/dt"
  Integrator/1 -> motor_rate_act/1, Add/2  "x"
  motorT/1 -> Divide/2

== system Model/Motor Model/MotorNonlinearDynamic5/Motor_Dynamics ==
  motor_rate_d : Inport
  ModelInit_RPM : Inport  Port=2
  motorT : Inport  Port=3
  Add : Sum  Inputs=+-
  Divide : Product  Inputs=*/
  Integrator : Integrator  InitialConditionSource=external
  motor_rate_act : Outport  VectorParamsAs1DForOutWhenUnconnected=off
  wires:
  motorT/1 -> Divide/2
  Integrator/1 -> Add/2, motor_rate_act/1  "x"
  Divide/1 -> Integrator/1  "drate/dt"
  motor_rate_d/1 -> Add/1
  ModelInit_RPM/1 -> Integrator/2
  Add/1 -> Divide/1

== system Model/Motor Model/MotorNonlinearDynamic6/Motor_Dynamics ==
  motor_rate_d : Inport
  ModelInit_RPM : Inport  Port=2
  motorT : Inport  Port=3
  Add : Sum  Inputs=+-
  Divide : Product  Inputs=*/
  Integrator : Integrator  InitialConditionSource=external
  motor_rate_act : Outport  VectorParamsAs1DForOutWhenUnconnected=off
  wires:
  Add/1 -> Divide/1
  ModelInit_RPM/1 -> Integrator/2
  motor_rate_d/1 -> Add/1
  Divide/1 -> Integrator/1  "drate/dt"
  Integrator/1 -> motor_rate_act/1, Add/2  "x"
  motorT/1 -> Divide/2

== system Model/Motor Model/MotorNonlinearDynamic7/Motor_Dynamics ==
  motor_rate_d : Inport
  ModelInit_RPM : Inport  Port=2
  motorT : Inport  Port=3
  Add : Sum  Inputs=+-
  Divide : Product  Inputs=*/
  Integrator : Integrator  InitialConditionSource=external
  motor_rate_act : Outport  VectorParamsAs1DForOutWhenUnconnected=off
  wires:
  motorT/1 -> Divide/2
  Integrator/1 -> Add/2, motor_rate_act/1  "x"
  Divide/1 -> Integrator/1  "drate/dt"
  motor_rate_d/1 -> Add/1
  ModelInit_RPM/1 -> Integrator/2
  Add/1 -> Divide/1

== system Model/Motor Model/MotorNonlinearDynamic8/Motor_Dynamics ==
  motor_rate_d : Inport
  ModelInit_RPM : Inport  Port=2
  motorT : Inport  Port=3
  Add : Sum  Inputs=+-
  Divide : Product  Inputs=*/
  Integrator : Integrator  InitialConditionSource=external
  motor_rate_act : Outport  VectorParamsAs1DForOutWhenUnconnected=off
  wires:
  Add/1 -> Divide/1
  ModelInit_RPM/1 -> Integrator/2
  motor_rate_d/1 -> Add/1
  Divide/1 -> Integrator/1  "drate/dt"
  Integrator/1 -> motor_rate_act/1, Add/2  "x"
  motorT/1 -> Divide/2

== system Model/SensorModel1/HILGPSModel/GyroNoiseSwitch2 ==
  In1 : Inport
  Constant1 : Constant  Value=ModelParam_GlobalNoiseGainSwitch
  Constant2 : Constant  Value=0.3
  Gain2 : Gain  Gain=0.7
  Product4 : Product
  Sum : Sum  Inputs=|++
  Out1 : Outport  VectorParamsAs1DForOutWhenUnconnected=off
  wires:
  Sum/1 -> Product4/2
  Product4/1 -> Out1/1
  Gain2/1 -> Sum/1
  In1/1 -> Product4/1
  Constant1/1 -> Gain2/1
  Constant2/1 -> Sum/2

== system Model/SensorModel1/HILGPSModel/NoiseFilter1 ==
  In1 : Inport
  Demux : Demux  Outputs=3
  Mux1 : Mux  Inputs=3
  Transfer Fcn1 : TransferFcn  Denominator=[0.05 1]
  Transfer Fcn2 : TransferFcn  Denominator=[0.05 1]
  Transfer Fcn4 : TransferFcn  Denominator=[0.05 1]
  Out1 : Outport  VectorParamsAs1DForOutWhenUnconnected=off
  wires:
  Mux1/1 -> Out1/1
  In1/1 -> Demux/1
  Demux/3 -> Transfer Fcn2/1
  Transfer Fcn4/1 -> Mux1/1
  Transfer Fcn2/1 -> Mux1/3
  Demux/1 -> Transfer Fcn4/1
  Transfer Fcn1/1 -> Mux1/2
  Demux/2 -> Transfer Fcn1/1

== system Model/SensorModel1/HILGPSModel/NoiseFilter2 ==
  In1 : Inport
  Demux : Demux  Outputs=3
  Mux1 : Mux  Inputs=3
  Transfer Fcn1 : TransferFcn  Denominator=[0.05 1]
  Transfer Fcn2 : TransferFcn  Denominator=[0.05 1]
  Transfer Fcn4 : TransferFcn  Denominator=[0.05 1]
  Out1 : Outport  VectorParamsAs1DForOutWhenUnconnected=off
  wires:
  Mux1/1 -> Out1/1
  In1/1 -> Demux/1
  Demux/3 -> Transfer Fcn2/1
  Transfer Fcn4/1 -> Mux1/1
  Transfer Fcn2/1 -> Mux1/3
  Demux/1 -> Transfer Fcn4/1
  Transfer Fcn1/1 -> Mux1/2
  Demux/2 -> Transfer Fcn1/1

== system Model/SensorModel1/HILGPSModel/Subsystem ==
  u : Inport
  Constant : Constant  Value=0
  Constant1 : Constant  Value=360
  Demux1 : Demux  Outputs=3
  Product : Product
  Product1 : Product
  Sqrt : Sqrt  SaturateOnIntegerOverflow=on
  Sum1 : Sum  Inputs=|++
  Sum4 : Sum  Inputs=|++
  Switch : Switch  Threshold=1
  Switch1 : Switch
  Terminator : Terminator
  Trigonometric Function : Trigonometry  Operator=atan2
  v : Outport  VectorParamsAs1DForOutWhenUnconnected=off
  cot : Outport  Port=2  VectorParamsAs1DForOutWhenUnconnected=off
  wires:
  Demux1/2 -> Trigonometric Function/2, Product1/2, Product1/1
  Product/1 -> Sum4/1
  u/1 -> Demux1/1
  Switch/1 -> Sum1/1, Switch1/1, Switch1/2
  Product1/1 -> Sum4/2
  Demux1/3 -> Terminator/1
  Sqrt/1 -> v/1, Switch/2
  Constant/1 -> Switch/3
  Trigonometric Function/1 -> Switch/1
  Sum4/1 -> Sqrt/1
  Demux1/1 -> Trigonometric Function/1, Product/1, Product/2
  Constant1/1 -> Sum1/2
  Sum1/1 -> Switch1/3
  Switch1/1 -> cot/1

== system Model/SensorModel1/HILGPSModel1/GyroNoiseSwitch2 ==
  In1 : Inport
  Constant1 : Constant  Value=ModelParam_GlobalNoiseGainSwitch
  Constant2 : Constant  Value=0.3
  Gain2 : Gain  Gain=0.7
  Product4 : Product
  Sum : Sum  Inputs=|++
  Out1 : Outport  VectorParamsAs1DForOutWhenUnconnected=off
  wires:
  Sum/1 -> Product4/2
  Product4/1 -> Out1/1
  Gain2/1 -> Sum/1
  In1/1 -> Product4/1
  Constant1/1 -> Gain2/1
  Constant2/1 -> Sum/2

== system Model/SensorModel1/HILGPSModel1/NoiseFilter1 ==
  In1 : Inport
  Demux : Demux  Outputs=3
  Mux1 : Mux  Inputs=3
  Transfer Fcn1 : TransferFcn  Denominator=[0.05 1]
  Transfer Fcn2 : TransferFcn  Denominator=[0.05 1]
  Transfer Fcn4 : TransferFcn  Denominator=[0.05 1]
  Out1 : Outport  VectorParamsAs1DForOutWhenUnconnected=off
  wires:
  Mux1/1 -> Out1/1
  In1/1 -> Demux/1
  Demux/3 -> Transfer Fcn2/1
  Transfer Fcn4/1 -> Mux1/1
  Transfer Fcn2/1 -> Mux1/3
  Demux/1 -> Transfer Fcn4/1
  Transfer Fcn1/1 -> Mux1/2
  Demux/2 -> Transfer Fcn1/1

== system Model/SensorModel1/HILGPSModel1/Subsystem ==
  u : Inport
  Constant : Constant  Value=0  SampleTime=Ts
  Constant1 : Constant  Value=360  SampleTime=Ts
  Demux1 : Demux  Outputs=3
  Product : Product
  Product1 : Product
  Sqrt : Sqrt  SaturateOnIntegerOverflow=on
  Sum1 : Sum  Inputs=|++
  Sum4 : Sum  Inputs=|++
  Switch : Switch  Threshold=1
  Switch1 : Switch
  Terminator : Terminator
  Trigonometric Function : Trigonometry  Operator=atan2
  v : Outport  VectorParamsAs1DForOutWhenUnconnected=off
  cot : Outport  Port=2  VectorParamsAs1DForOutWhenUnconnected=off
  wires:
  Demux1/2 -> Trigonometric Function/2, Product1/2, Product1/1
  Product/1 -> Sum4/1
  u/1 -> Demux1/1
  Switch/1 -> Sum1/1, Switch1/1, Switch1/2
  Product1/1 -> Sum4/2
  Demux1/3 -> Terminator/1
  Sqrt/1 -> v/1, Switch/2
  Constant/1 -> Switch/3
  Trigonometric Function/1 -> Switch/1
  Sum4/1 -> Sqrt/1
  Demux1/1 -> Trigonometric Function/1, Product/1, Product/2
  Constant1/1 -> Sum1/2
  Sum1/1 -> Switch1/3
  Switch1/1 -> cot/1

== system Model/SensorModel1/HILSensorMavModel1/GyroNoiseSwitch0 ==
  In1 : Inport
  Constant1 : Constant  Value=ModelParam_GlobalNoiseGainSwitch
  Constant2 : Constant  Value=0.2
  Gain2 : Gain  Gain=0.8
  Product4 : Product
  Sum : Sum  Inputs=|++
  Out1 : Outport  VectorParamsAs1DForOutWhenUnconnected=off
  wires:
  Sum/1 -> Product4/2
  Product4/1 -> Out1/1
  Gain2/1 -> Sum/1
  In1/1 -> Product4/1
  Constant1/1 -> Gain2/1
  Constant2/1 -> Sum/2

== system Model/SensorModel1/HILSensorMavModel1/GyroNoiseSwitch1 ==
  In1 : Inport
  Constant1 : Constant  Value=ModelParam_GlobalNoiseGainSwitch
  Constant2 : Constant  Value=0.2
  Gain2 : Gain  Gain=0.8
  Product4 : Product
  Sum : Sum  Inputs=|++
  Out1 : Outport  VectorParamsAs1DForOutWhenUnconnected=off
  wires:
  Sum/1 -> Product4/2
  Product4/1 -> Out1/1
  Gain2/1 -> Sum/1
  In1/1 -> Product4/1
  Constant1/1 -> Gain2/1
  Constant2/1 -> Sum/2

== system Model/SensorModel1/HILSensorMavModel1/GyroNoiseSwitch2 ==
  In1 : Inport
  Constant1 : Constant  Value=ModelParam_GlobalNoiseGainSwitch
  Constant2 : Constant  Value=0.2
  Gain2 : Gain  Gain=0.8
  Product4 : Product
  Sum : Sum  Inputs=|++
  Out1 : Outport  VectorParamsAs1DForOutWhenUnconnected=off
  wires:
  Sum/1 -> Product4/2
  Product4/1 -> Out1/1
  Gain2/1 -> Sum/1
  In1/1 -> Product4/1
  Constant1/1 -> Gain2/1
  Constant2/1 -> Sum/2

== system Model/SensorModel1/HILSensorMavModel1/GyroNoiseSwitch3 ==
  In1 : Inport
  Constant1 : Constant  Value=ModelParam_GlobalNoiseGainSwitch
  Constant2 : Constant  Value=0.3
  Gain2 : Gain  Gain=0.7
  Product4 : Product
  Sum : Sum  Inputs=|++
  Out1 : Outport  VectorParamsAs1DForOutWhenUnconnected=off
  wires:
  Sum/1 -> Product4/2
  Product4/1 -> Out1/1
  Gain2/1 -> Sum/1
  In1/1 -> Product4/1
  Constant1/1 -> Gain2/1
  Constant2/1 -> Sum/2

== system Model/SensorModel1/HILSensorMavModel1/GyroNoiseSwitch4 ==
  In1 : Inport
  Constant1 : Constant  Value=ModelParam_GlobalNoiseGainSwitch
  Constant2 : Constant  Value=0.3
  Gain2 : Gain  Gain=0.7
  Product4 : Product
  Sum : Sum  Inputs=|++
  Out1 : Outport  VectorParamsAs1DForOutWhenUnconnected=off
  wires:
  Sum/1 -> Product4/2
  Product4/1 -> Out1/1
  Gain2/1 -> Sum/1
  In1/1 -> Product4/1
  Constant1/1 -> Gain2/1
  Constant2/1 -> Sum/2

== stateflow chart Model/Chart ==
  settings: executeAtInitialization=1
  state idle
    entry:S = 1;
    Accel_Mag = 0;
    status = 0;
    step = 1;
  state runningModel
    entry:Accel_Mag = 0;
    status = 0;
    S = 1;
  state CalMag
    entry:S = 0;
    Accel_Mag = 1;
    status = 2;
  state CalAccel
    entry:S = 0;
    Accel_Mag = 0;
    status = 1;
  (default) -> idle
  idle -> runningModel : [mod==false&stepUp ==false]{step = 1;}
  CalMag -> runningModel [order 1] : [mod]{step = 1;}
  runningModel -> CalAccel : [mod]{step = 1;}
  CalMag -> CalMag [order 2] : [stepUp]{step = min(step +1,18);}
  CalAccel -> CalMag [order 1] : [mod==1]{step = 1;}
  CalAccel -> CalAccel [order 2] : [stepUp]{step = min(step +1,8);}
  data: mod input boolean size=1; stepUp input boolean size=1; S output uint8 size=1; Accel_Mag output uint8 size=1; step output uint8 size=1; status output uint8 size=1
